simulink model "Modelo_Anfis_Directo"  (R2019a)
settings: Solver=VariableStepAuto  StartTime=0.0  StopTime=600  RelTol=1e-3
values from neighbouring files (symbols this model uses):
  Tm = 0.6    [ANFIS_inverso.m]    (also in Codigo_Inverso.m; Codigo_directo.m = 0.2)
libraries: fuzblock x1
settings Model: Creator=Jose  LastModifiedBy=Jose

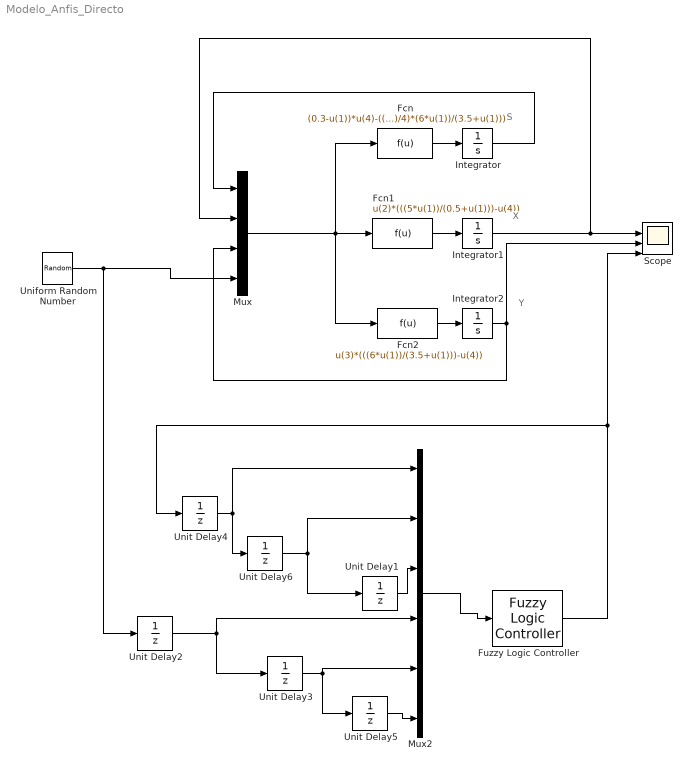
== system Modelo_Anfis_Directo ==
  note: Y
  note: S
  note: X
  Fcn : Fcn  Expr=(0.3-u(1))*u(4)-((u(2)/4)*(5*u(1))/(0.5+u(1)))-((u(3)/4)*(6*u(1))/(3.5+u(1)))
  Fcn1 : Fcn  Expr=u(2)*(((5*u(1))/(0.5+u(1)))-u(4))
  Fcn2 : Fcn  Expr=u(3)*(((6*u(1))/(3.5+u(1)))-u(4))
  Fuzzy Logic Controller : fuzblock/Fuzzy Logic  Controller  FIS=fis  OutputSampleNumber=101  DataType=double  FuzzifiedInputs=off  RuleFiringStrengths=off  RuleOutputs=off  AggregatedOutputs=off  SimulateUsing=Interpreted execution  OutOfRangeInputValueMessage=warning  NoRuleFiredMessage=warning  EmptyOutputFuzzySetMessage=warning
  Integrator : Integrator
  Integrator1 : Integrator  InitialCondition=0.1
  Integrator2 : Integrator
  Mux : Mux
  Mux2 : Mux  Inputs=6
  Scope : Scope  NumInputPorts=4
  Uniform Random Number : UniformRandomNumber  Minimum=0.1  Maximum=1.7  Seed=456  SampleTime=60
  Unit Delay{1..6} (6 alike) : UnitDelay  SampleTime=Tm  HasFrameUpgradeWarning=on
  wires:
  Integrator1/1 -> Mux/2, Scope/2
  Fcn2/1 -> Integrator2/1
  Mux/1 -> Fcn/1, Fcn1/1, Fcn2/1
  Integrator2/1 -> Mux/3, Scope/3
  Fcn/1 -> Integrator/1
  Integrator/1 -> Mux/1
  Fcn1/1 -> Integrator1/1
  Fuzzy Logic Controller/1 -> Unit Delay4/1, Scope/4
  Unit Delay5/1 -> Mux2/6
  Unit Delay4/1 -> Mux2/1, Unit Delay6/1
  Unit Delay1/1 -> Mux2/3
  Mux2/1 -> Fuzzy Logic Controller/1
  Unit Delay3/1 -> Mux2/5, Unit Delay5/1
  Uniform Random Number/1 -> Mux/4, Unit Delay2/1
  Unit Delay6/1 -> Mux2/2, Unit Delay1/1
  Unit Delay2/1 -> Mux2/4, Unit Delay3/1
